simulink model "ex4_step7"  (R2016b)
settings: Solver=VariableStepAuto  StartTime=0.0  StopTime=10.0  RelTol=1e-3
settings Model: Creator=drazz  LastModifiedBy=drazz

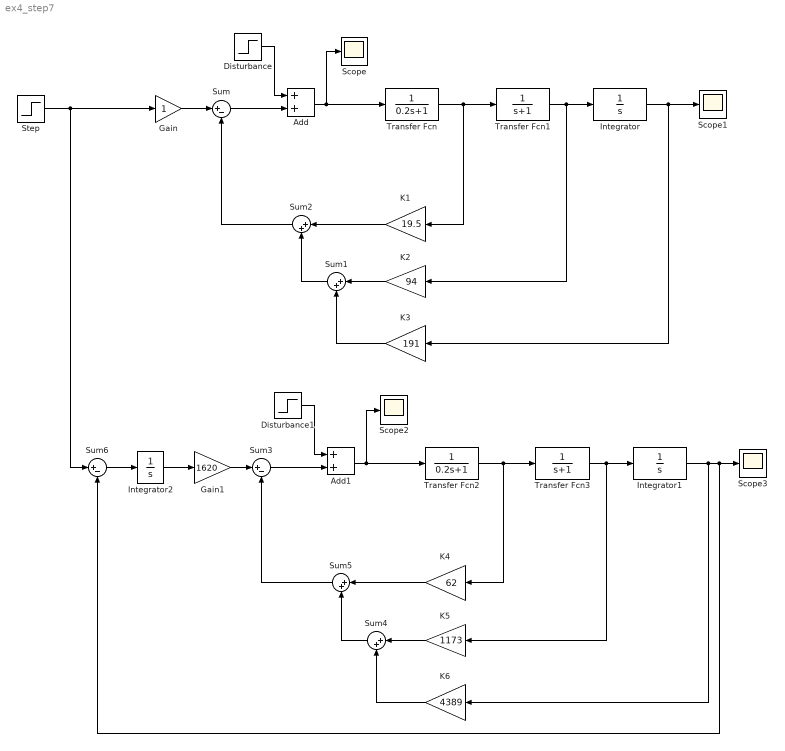
== system ex4_step7 ==
  Add : Sum
  Add1 : Sum
  Disturbance : Step  SampleTime=0
  Disturbance1 : Step  SampleTime=0
  Gain : Gain
  Gain1 : Gain  Gain=1620
  Integrator : TransferFcn  Denominator=[1 0]
  Integrator1 : TransferFcn  Denominator=[1 0]
  Integrator2 : TransferFcn  Denominator=[1 0]
  K1 : Gain  Gain=19.5
  K2 : Gain  Gain=94
  K3 : Gain  Gain=191
  K4 : Gain  Gain=62
  K5 : Gain  Gain=1173
  K6 : Gain  Gain=4389
  Scope{,1..3} (4 alike) : Scope
  Step : Step  SampleTime=0
  Sum : Sum  Inputs=|+-
  Sum{1..2,4..5} (4 alike) : Sum  Inputs=|++
  Sum3 : Sum  Inputs=|+-
  Sum6 : Sum  Inputs=|+-
  Transfer Fcn : TransferFcn  Denominator=[0.2 1]
  Transfer Fcn1 : TransferFcn  Denominator=[1 1]
  Transfer Fcn2 : TransferFcn  Denominator=[0.2 1]
  Transfer Fcn3 : TransferFcn  Denominator=[1 1]
  wires:
  Add/1 -> Transfer Fcn/1, Scope/1
  Step/1 -> Gain/1, Sum6/1
  Gain/1 -> Sum/1
  Sum/1 -> Add/2
  Disturbance/1 -> Add/1
  Transfer Fcn/1 -> K1/1, Transfer Fcn1/1
  Transfer Fcn1/1 -> K2/1, Integrator/1
  Integrator/1 -> K3/1, Scope1/1
  K1/1 -> Sum2/1
  K2/1 -> Sum1/1
  K3/1 -> Sum1/2
  Sum1/1 -> Sum2/2
  Sum2/1 -> Sum/2
  Add1/1 -> Transfer Fcn2/1, Scope2/1
  Gain1/1 -> Sum3/1
  Sum3/1 -> Add1/2
  Disturbance1/1 -> Add1/1
  Transfer Fcn2/1 -> K4/1, Transfer Fcn3/1
  Transfer Fcn3/1 -> K5/1, Integrator1/1
  Integrator1/1 -> K6/1, Sum6/2, Scope3/1
  K4/1 -> Sum5/1
  K5/1 -> Sum4/1
  K6/1 -> Sum4/2
  Sum4/1 -> Sum5/2
  Sum5/1 -> Sum3/2
  Integrator2/1 -> Gain1/1
  Sum6/1 -> Integrator2/1
